simulink model "slm1"  (R2018a)
settings: Solver=VariableStepAuto  StartTime=0.0  StopTime=10.0  RelTol=1e-3
values from neighbouring files (symbols this model uses):
  F = 10    [setup.m]
  k = [.1,1,5]    [setup.m]
settings Model: Creator=Pranav Maddula  LastModifiedBy=Pranav Maddula

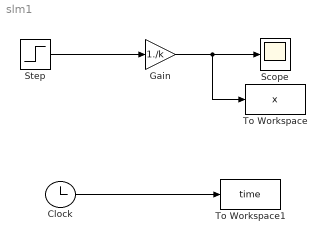
== system slm1 ==
  Clock : Clock
  Gain : Gain  Gain=1./k
  Scope : Scope
  Step : Step  After=F  SampleTime=0
  To Workspace : ToWorkspace  VariableName=x  SampleTime=-1
      settings: Save2DSignal=2-D array (concatenate along first dimension)
  To Workspace1 : ToWorkspace  VariableName=time  SampleTime=-1
      settings: Save2DSignal=2-D array (concatenate along first dimension)
  wires:
  Step/1 -> Gain/1
  Gain/1 -> To Workspace/1, Scope/1
  Clock/1 -> To Workspace1/1
